simulink model "ode_sine"  (R2023a)
settings: Solver=FixedStepAuto  StartTime=0.0  StopTime=100  FixedStep=0.01  RelTol=1e-3
settings Model: Creator=junho  LastModifiedBy=junho

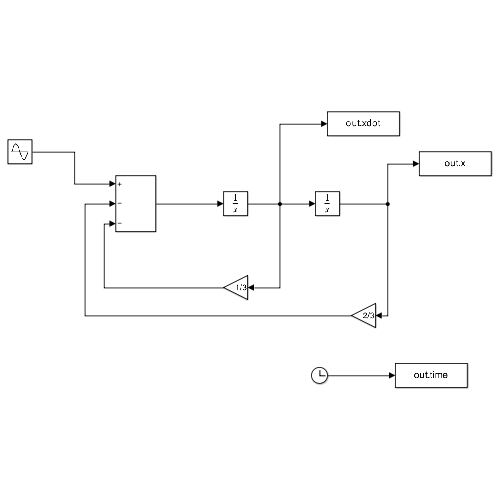
[thumbnail: Simulink's stored preview of the top-level diagram]
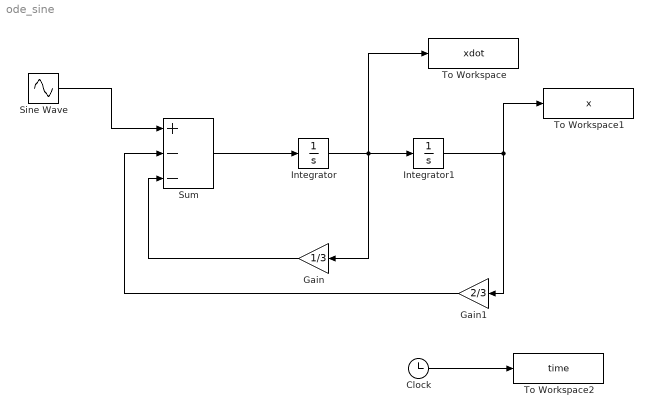
== system ode_sine ==
  Clock : Clock
  Gain : Gain  Gain=1/3
  Gain1 : Gain  Gain=2/3
  Integrator : Integrator
  Integrator1 : Integrator
  Sine Wave : Sin  SampleTime=0
  Sum : Sum  Inputs=+--
  To Workspace : ToWorkspace  VariableName=xdot  SampleTime=-1
  To Workspace1 : ToWorkspace  VariableName=x  SampleTime=-1
  To Workspace2 : ToWorkspace  VariableName=time  SampleTime=-1
  wires:
  Sum/1 -> Integrator/1
  Integrator/1 -> To Workspace/1, Integrator1/1, Gain/1
  Gain/1 -> Sum/3
  Integrator1/1 -> To Workspace1/1, Gain1/1
  Gain1/1 -> Sum/2
  Sine Wave/1 -> Sum/1
  Clock/1 -> To Workspace2/1
